simulink model "final"  (R2019a)
settings: Solver=ode45  StartTime=0.0  StopTime=3  RelTol=1e-3  EnableMultiTasking=on
undefined symbols (not defined in the file): FZ_alpha_final, FZ_K1_final, FZ_Ke_final, Ki, Kp, Omega_d_max
libraries: fuzblock x1, simulink x1
settings Model: Creator=Stelios  LastModifiedBy=Thanasis Charisoudis
settings DataIOCC: LimitDataPoints=on  SaveFormat=Array  InspectSignalLogs=on  ReturnWorkspaceOutputs=off
settings OptimizationCC: LifeSpan=inf
settings DebuggingCC: SFUnexpectedBacktrackingDiag=warning  SFNoUnconditionalDefaultTransitionDiag=warning  SFExecutionAtInitializationDiag=none  ArithmeticOperatorsInVariantConditions=warning
settings HardwareCC: ProdBitPerPointer=32  ProdBitPerSizeT=32  ProdBitPerPtrDiffT=32  ProdLargestAtomicFloat=None  ProdIntDivRoundTo=Undefined  ProdEndianess=Unspecified  ProdWordSize=32  ProdHWDeviceType=32-bit Generic
settings ModelReferenceCC: PropagateSignalLabelsOutOfModel=off
settings SFSimCC: SimUseLocalCustomCode=off
settings RTWCC: RTWUseLocalCustomCode=off
settings CodeAppCC: StateflowObjectComments=on
settings GRTTargetCC: TargetLangStandard=C89/C90 (ANSI)  GeneratePreprocessorConditionals=Disable all
settings ConfigComp: CovMetricSettings=dw  CovHtmlReporting=on  CovSaveCumulativeToWorkspaceVar=on  CovSaveSingleToWorkspaceVar=on  CovExternalEMLEnable=off

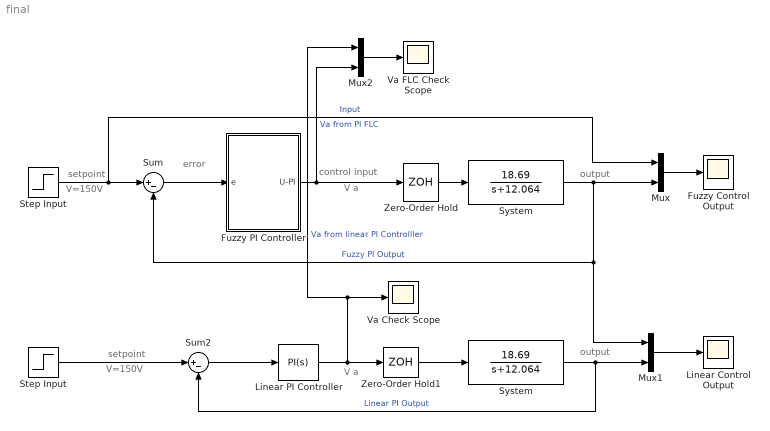
== system final ==
  note: setpoint
  note: output
  note: error
  note: control input
  note: V a
  note: V=150V
  note: setpoint
  note: V=150V
  note: V a
  note: output
  Fuzzy Control Output : Scope
  Fuzzy PI Controller : Subsystem
  Linear Control Output : Scope
  Linear PI Controller : simulink/Continuous/PID Controller  Controller=PI  Form=Parallel  TimeDomain=Continuous-time  SampleTime=0.01  IntegratorMethod=Forward Euler  FilterMethod=Forward Euler  ControllerParametersSource=internal  P=Kp  I=Ki  D=0  UseFilter=on  N=100  TunerSelectOption=Transfer Function Based (PID Tuner App)  InitialConditionSource=internal  InitialConditionForIntegrator=0  InitialConditionForFilter=0  DifferentiatorICPrevScaledInput=0  ExternalReset=none  TrackingMode=off  Kt=1  LimitOutput=off  UpperSaturationLimit=inf  LowerSaturationLimit=-inf  LinearizeAsGain=on  AntiWindupMode=none  Kb=1  RndMeth=Round  POutMin=[]  POutMax=[]  IOutMin=[]  IOutMax=[]  DOutMin=[]  DOutMax=[]  NOutMin=[]  NOutMax=[]  SumOutMin=[]  SumOutMax=[]  SaturationOutMin=[]  SaturationOutMax=[]  PParamMin=[]  PParamMax=[]  IParamMin=[]  IParamMax=[]  DParamMin=[]  DParamMax=[]  NParamMin=[]  NParamMax=[]  KbParamMin=[]  KbParamMax=[]  KtParamMin=[]  KtParamMax=[]  KbOutMin=[]  KbOutMax=[]  KtOutMin=[]  KtOutMax=[]  IntegratorOutMin=[]  IntegratorOutMax=[]  FilterOutMin=[]  FilterOutMax=[]  SumI1OutMin=[]  SumI1OutMax=[]  SumI2OutMin=[]  SumI2OutMax=[]  SumI3OutMin=[]  SumI3OutMax=[]  SumI4OutMin=[]  SumI4OutMax=[]  SumDOutMin=[]  SumDOutMax=[]  DifferentiatorOutMin=[]  DifferentiatorOutMax=[]  FilterDiffOutCoefMin=[]  FilterDiffOutCoefMax=[]  ReciprocalOutMin=[]  ReciprocalOutMax=[]  SumDenOutMin=[]  SumDenOutMax=[]  SumNumOutMin=[]  SumNumOutMax=[]  DivideOutMin=[]  DivideOutMax=[]  IntegratorContinuousStateAttributes=''  IntegratorStateMustResolveToSignalObject=off  IntegratorRTWStateStorageClass=Auto  FilterContinuousStateAttributes=''  FilterStateMustResolveToSignalObject=off  FilterRTWStateStorageClass=Auto  ParallelPVariant=InternalParameters  IdealPVariant=Disabled  IVariant=InternalParameters  DVariant=Disabled  IntegratorVariant=Continuous  SatVariant=Disabled  AWVariant=Passthrough  PCopyVariant=Disabled  TRVariant=Disabled  FdbkBlocksVariant=Forward  IdealPFdbkVariant=Disabled  SatFdbkVariant=Disabled  DerivativeFilterVariant=Disabled  NVariant=Disabled  NCopyVariant=Disabled_SignalSpec  FilterICVariant=Disabled  IntegratorICVariant=InternalICs  ExternalResetVariant=Disabled  TRSumVariant=Passthrough  SumFdbkVariant=Disabled  SumVariant=Sum_PI
  Mux : Mux  Inputs=2
  Mux1 : Mux  Inputs=2
  Mux2 : Mux  Inputs=2
  Step Input : Step  Time=0  After=Omega_d_max  SampleTime=0.1
  "Step Input " : Step  Time=0  After=Omega_d_max  SampleTime=0.1
  Sum : Sum  Inputs=|+-  SaturateOnIntegerOverflow=on
  Sum2 : Sum  Inputs=|+-
  System : TransferFcn  Numerator=[18.69]  Denominator=[1 12.064]
  "System " : TransferFcn  Numerator=[18.69]  Denominator=[1 12.064]
  Va Check Scope : Scope
  Va FLC Check Scope : Scope
  Zero-Order Hold : ZeroOrderHold  SampleTime=0.01
  Zero-Order Hold1 : ZeroOrderHold  SampleTime=0.01
  wires:
  Sum/1 -> Fuzzy PI Controller/1(e)
  Fuzzy PI Controller/1(U-PI) -> Mux2/2, Zero-Order Hold/1  "Va from PI FLC"
  Zero-Order Hold/1 -> System/1
  Mux/1 -> Fuzzy Control Output/1
  System/1 -> Mux/2, Mux1/1, Sum/2  "Fuzzy PI Output"
  Mux1/1 -> Linear Control Output/1
  Linear PI Controller/1 -> Mux2/1, Va Check Scope/1, Zero-Order Hold1/1  "Va from linear PI Controlller"
  Sum2/1 -> Linear PI Controller/1
  "Step Input "/1 -> Sum/1, Mux/1  "Input"
  Step Input/1 -> Sum2/1
  Zero-Order Hold1/1 -> "System "/1
  "System "/1 -> Mux1/2, Sum2/2  "Linear PI Output"
  Mux2/1 -> Va FLC Check Scope/1

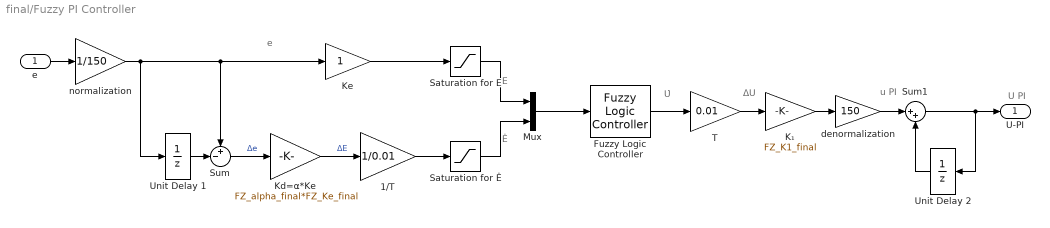
== system final/Fuzzy PI Controller ==
  note: e
  note: E
  note: Ė
  note: U̇
  note: ΔU
  note: u PI
  note: U PI
  e : Inport
  1/T : Gain  Gain=1/0.01  SaturateOnIntegerOverflow=on  OutDataTypeStr=Inherit: Same as input  ParamDataTypeStr=Inherit: Same as input
  Fuzzy Logic Controller : fuzblock/Fuzzy Logic  Controller  FIS='fuzzy_rule_base.fis'  OutputSampleNumber=101  DataType=double  FuzzifiedInputs=off  RuleFiringStrengths=off  RuleOutputs=off  AggregatedOutputs=off  SimulateUsing=Interpreted execution  OutOfRangeInputValueMessage=warning  NoRuleFiredMessage=warning  EmptyOutputFuzzySetMessage=warning
  Kd=α*Ke : Gain  Gain=FZ_alpha_final*FZ_Ke_final  SaturateOnIntegerOverflow=on  OutDataTypeStr=Inherit: Same as input  ParamDataTypeStr=Inherit: Same as input
  Ke : Gain  SaturateOnIntegerOverflow=on  OutDataTypeStr=Inherit: Same as input  ParamDataTypeStr=Inherit: Same as input
  K₁ : Gain  Gain=FZ_K1_final  SaturateOnIntegerOverflow=on  OutDataTypeStr=Inherit: Same as input  ParamDataTypeStr=Inherit: Same as input
  Mux : Mux  Inputs=2
  Saturation for Ė : Saturate  UpperLimit=1  LowerLimit=-1
  Saturation for Ε : Saturate  UpperLimit=1  LowerLimit=-1
  Sum : Sum  Inputs=+-|  SaturateOnIntegerOverflow=on
  Sum1 : Sum  Inputs=|++  SaturateOnIntegerOverflow=on
  T : Gain  Gain=0.01  SaturateOnIntegerOverflow=on  OutDataTypeStr=Inherit: Same as input  ParamDataTypeStr=Inherit: Same as input
  Unit Delay 1 : UnitDelay  SampleTime=0.01  HasFrameUpgradeWarning=on
  Unit Delay 2 : UnitDelay  SampleTime=0.01  HasFrameUpgradeWarning=on
  denormalization : Gain  Gain=150  SaturateOnIntegerOverflow=on  OutDataTypeStr=Inherit: Same as input  ParamDataTypeStr=Inherit: Same as input
  normalization : Gain  Gain=1/150  SaturateOnIntegerOverflow=on  OutDataTypeStr=Inherit: Same as input  ParamDataTypeStr=Inherit: Same as input
  U-PI : Outport
  wires:
  e/1 -> normalization/1
  normalization/1 -> Unit Delay 1/1, Ke/1, Sum/1
  Ke/1 -> Saturation for Ε/1
  Saturation for Ε/1 -> Mux/1
  Fuzzy Logic Controller/1 -> T/1
  T/1 -> K₁/1
  K₁/1 -> denormalization/1
  denormalization/1 -> Sum1/1
  Sum1/1 -> U-PI/1, Unit Delay 2/1
  Unit Delay 2/1 -> Sum1/2
  Unit Delay 1/1 -> Sum/2
  Sum/1 -> Kd=α*Ke/1  "Δe"
  Kd=α*Ke/1 -> 1/T/1  "ΔE"
  1/T/1 -> Saturation for Ė/1
  Saturation for Ė/1 -> Mux/2
  Mux/1 -> Fuzzy Logic Controller/1
